simulink model "qp_torq_allocator"  (R2024b)
settings: Solver=VariableStepAuto  StartTime=0.0  StopTime=10.0  RelTol=1e-3
settings Model: Creator=lukec  LastModifiedBy=lukec

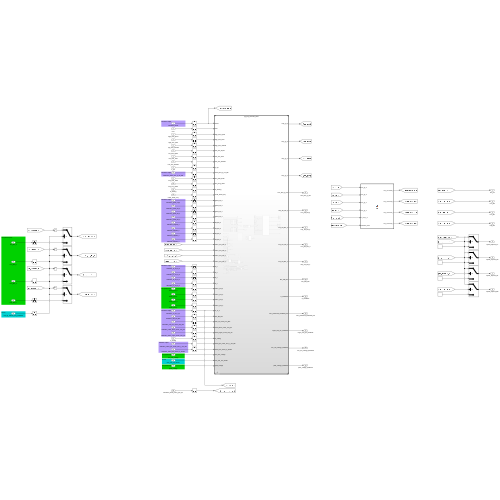
[thumbnail: Simulink's stored preview of the top-level diagram]
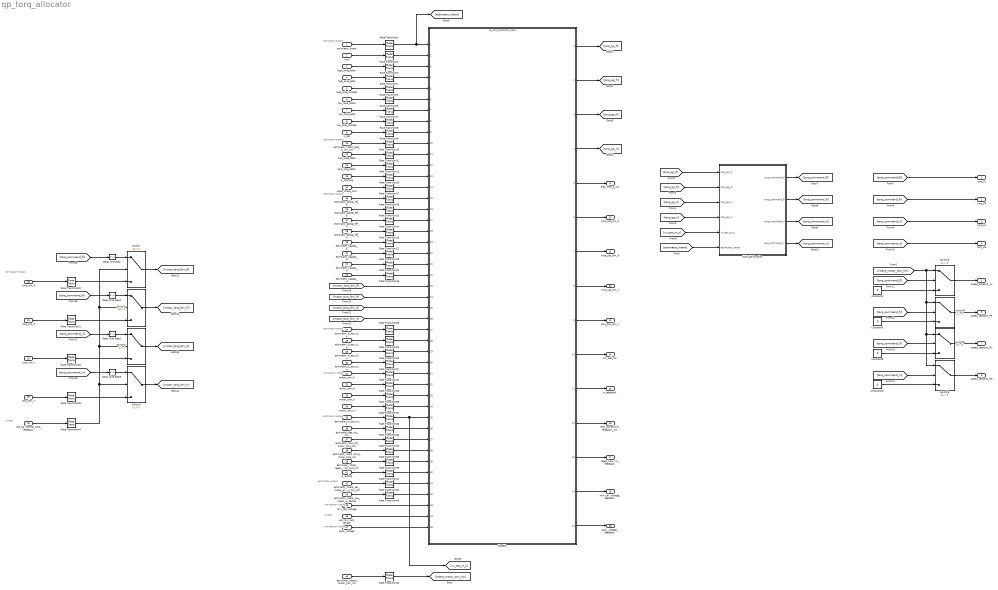
== system qp_torq_allocator ==
  note: non-param-inputs
  note: estimator-output
  note: estimator-output
  note: non-param-inputs
  note: estimator-output
  note: estimator-output
  note: estimator-output
  note: estimator-output
  note: is-bool
  note: non-param-inputs
  note: is-bool
  note: non-param-inputs
  estimator_intent : Inport
  mux : Inport  Port=2
  high_axle_alpha : Inport  Port=3
  high_axle_beta : Inport  Port=4
  high_axle_lambda : Inport  Port=5
  low_axle_alpha : Inport  Port=6
  low_axle_beta : Inport  Port=7
  low_axle_lambda : Inport  Port=8
  k_opt : Inport  Port=9
  estimator_intent_elec_p_lim_kW : Inport  Port=10
  torq_side_delta : Inport  Port=11
  torq_long_delta : Inport  Port=12
  w_starting : Inport  Port=13
  coast_brake_torq : Inport  Port=14
  estimator_global_eff_fl : Inport  Port=15
  estimator_global_eff_fr : Inport  Port=16
  estimator_global_eff_rl : Inport  Port=17
  estimator_global_eff_rr : Inport  Port=18
  estimator_kappas_fl : Inport  Port=19
  estimator_kappas_fr : Inport  Port=20
  estimator_kappas_rl : Inport  Port=21
  estimator_kappas_rr : Inport  Port=22
  torq_Nm_fl : Inport  Port=23
  torq_Nm_fr : Inport  Port=24
  torq_Nm_rl : Inport  Port=25
  torq_Nm_rr : Inport  Port=26
  estimator_fz_est_N_fl : Inport  Port=27
  estimator_fz_est_N_fr : Inport  Port=28
  estimator_fz_est_N_rl : Inport  Port=29
  estimator_fz_est_N_rr : Inport  Port=30
  motor_rpm_fl : Inport  Port=31
  motor_rpm_fr : Inport  Port=32
  motor_rpm_rl : Inport  Port=33
  motor_rpm_rr : Inport  Port=34
  estimator_vx_est_m_s : Inport  Port=35
  estimator_des_Mz_Nm : Inport  Port=36
  estimator_max_tot_motor_torq_Nm : Inport  Port=37
  estimator_intent_drive_motor_torq_lim : Inport  Port=38
  estimator_intent_regen_motor_torq_lim : Inport  Port=39
  estimator_intent_motor_rpm_lim : Inport  Port=40
  w_ending : Inport  Port=41
  estimator_intent_per_motor_elec_p_lim_kW : Inport  Port=42
  estimator_intent_use_intent_w_derate : Inport  Port=43
  use_qp_internal_torq_feedback : Inport  Port=44  OutDataTypeStr=boolean
  min_cell_voltage : Inport  Port=45
  use_min_cell_derate : Inport  Port=46  OutDataTypeStr=boolean
  pack_voltage : Inport  Port=47
  Constant{4,6,8,10} (4 alike) : Constant  Value=0
  Delay One Step{,1..3} (4 alike) : Delay  DelayLength=1  SampleTime=0.004
  MATLAB Function : MATLAB Function  TreatAsAtomicUnit=on
  Model5 : ModelReference  ModelNameDialog=qp_torq_allocator_base.slx  SimulationMode=Normal  ModelReferenceVersion=1.26
  Rate Transition{1..44} (44 alike) : RateTransition  OutPortSampleTime=0.004
  Switch{,1..7} (8 alike) : Switch  Criteria=u2 > Threshold  SaturateOnIntegerOverflow=off  InputSameDT=off
  torq_FL : Outport
  torq_FR : Outport  Port=2
  torq_RL : Outport  Port=3
  torq_RR : Outport  Port=4
  speed_setpoint_FL : Outport  Port=5
  speed_setpoint_FR : Outport  Port=6
  speed_setpoint_RL : Outport  Port=7
  speed_setpoint_RR : Outport  Port=8
  elec_theo_p_kW : Outport  Port=9
  torq_sat_Nm_fl : Outport  Port=10
  torq_sat_Nm_fr : Outport  Port=11
  torq_sat_Nm_rl : Outport  Port=12
  torq_sat_Nm_rr : Outport  Port=13
  Mz_add_Nm : Outport  Port=14
  w_feedback : Outport  Port=15
  elec_powerlimit_feedback_kW : Outport  Port=16
  regen_torq_lim_feedback : Outport  Port=17
  min_cell_voltage_feedback : Outport  Port=18
  pack_voltage_feedback : Outport  Port=19
  wires:
  estimator_intent/1 -> Rate Transition1/1
  mux/1 -> Rate Transition2/1
  high_axle_alpha/1 -> Rate Transition3/1
  high_axle_beta/1 -> Rate Transition4/1
  high_axle_lambda/1 -> Rate Transition5/1
  low_axle_alpha/1 -> Rate Transition6/1
  low_axle_beta/1 -> Rate Transition7/1
  low_axle_lambda/1 -> Rate Transition8/1
  k_opt/1 -> Rate Transition9/1
  estimator_intent_elec_p_lim_kW/1 -> Rate Transition10/1
  torq_side_delta/1 -> Rate Transition11/1
  torq_long_delta/1 -> Rate Transition12/1
  w_starting/1 -> Rate Transition16/1
  coast_brake_torq/1 -> Rate Transition17/1
  estimator_global_eff_fl/1 -> Rate Transition18/1
  estimator_global_eff_fr/1 -> Rate Transition13/1
  estimator_global_eff_rl/1 -> Rate Transition14/1
  estimator_global_eff_rr/1 -> Rate Transition15/1
  estimator_kappas_fl/1 -> Rate Transition22/1
  estimator_kappas_fr/1 -> Rate Transition23/1
  estimator_kappas_rl/1 -> Rate Transition24/1
  estimator_kappas_rr/1 -> Rate Transition19/1
  torq_Nm_fl/1 -> Rate Transition20/1
  torq_Nm_fr/1 -> Rate Transition21/1
  torq_Nm_rl/1 -> Rate Transition28/1
  torq_Nm_rr/1 -> Rate Transition29/1
  estimator_fz_est_N_fl/1 -> Rate Transition30/1
  estimator_fz_est_N_fr/1 -> Rate Transition25/1
  estimator_fz_est_N_rl/1 -> Rate Transition26/1
  estimator_fz_est_N_rr/1 -> Rate Transition27/1
  motor_rpm_fl/1 -> Rate Transition31/1
  motor_rpm_fr/1 -> Rate Transition35/1
  motor_rpm_rl/1 -> Rate Transition36/1
  motor_rpm_rr/1 -> Rate Transition37/1
  estimator_vx_est_m_s/1 -> Rate Transition32/1
  estimator_des_Mz_Nm/1 -> Rate Transition33/1
  estimator_max_tot_motor_torq_Nm/1 -> Rate Transition34/1
  estimator_intent_drive_motor_torq_lim/1 -> Rate Transition38/1
  estimator_intent_regen_motor_torq_lim/1 -> Rate Transition39/1
  Rate Transition1/1 -> [estimator_intent], Model5/1
  Rate Transition2/1 -> Model5/2
  Rate Transition3/1 -> Model5/3
  Rate Transition6/1 -> Model5/6
  Rate Transition5/1 -> Model5/5
  Rate Transition4/1 -> Model5/4
  Rate Transition8/1 -> Model5/8
  Rate Transition10/1 -> Model5/10
  Rate Transition11/1 -> Model5/11
  Rate Transition9/1 -> Model5/9
  Rate Transition12/1 -> Model5/12
  Rate Transition7/1 -> Model5/7
  Rate Transition14/1 -> Model5/17
  Rate Transition15/1 -> Model5/18
  Rate Transition16/1 -> Model5/13
  Rate Transition17/1 -> Model5/14
  Rate Transition13/1 -> Model5/16
  Rate Transition18/1 -> Model5/15
  Rate Transition19/1 -> Model5/22
  Rate Transition24/1 -> Model5/21
  Rate Transition22/1 -> Model5/19
  Rate Transition23/1 -> Model5/20
  Rate Transition26/1 -> Model5/29
  Rate Transition27/1 -> Model5/30
  Rate Transition30/1 -> Model5/27
  Rate Transition25/1 -> Model5/28
  Rate Transition31/1 -> Model5/31
  Rate Transition32/1 -> [vx_est_m_s], Model5/35
  Rate Transition33/1 -> Model5/36
  Rate Transition34/1 -> Model5/37
  Rate Transition35/1 -> Model5/32
  Rate Transition36/1 -> Model5/33
  Rate Transition37/1 -> Model5/34
  Rate Transition39/1 -> Model5/39
  Rate Transition38/1 -> Model5/38
  estimator_intent_motor_rpm_lim/1 -> Rate Transition40/1
  Rate Transition40/1 -> [intent_motor_rpm_lim]
  Model5/1 -> [torq_qp_fl]
  Model5/2 -> [torq_qp_fr]
  Model5/3 -> [torq_qp_rl]
  Model5/4 -> [torq_qp_rr]
  Constant8/1 -> Switch5/3
  Switch4/1 -> speed_setpoint_FR/1
  Switch3/1 -> speed_setpoint_FL/1
  [torq_command_fr] -> Switch4/2
  [intent_motor_rpm_lim] -> Switch6/1, Switch5/1, Switch4/1, Switch3/1
  Switch6/1 -> speed_setpoint_RR/1
  [torq_command_rr] -> Switch6/2
  Constant4/1 -> Switch3/3
  [torq_command_rl] -> Switch5/2
  Constant6/1 -> Switch4/3
  Constant10/1 -> Switch6/3
  [torq_command_fl] -> Switch3/2
  Switch5/1 -> speed_setpoint_RL/1
  Model5/5 -> elec_theo_p_kW/1
  Model5/6 -> torq_sat_Nm_fl/1
  Model5/7 -> torq_sat_Nm_fr/1
  Model5/8 -> torq_sat_Nm_rl/1
  Model5/9 -> torq_sat_Nm_rr/1
  Model5/10 -> Mz_add_Nm/1
  [torq_qp_fl] -> MATLAB Function/1(torq_qp_fl)
  [torq_qp_fr] -> MATLAB Function/2(torq_qp_fr)
  [torq_qp_rl] -> MATLAB Function/3(torq_qp_rl)
  [torq_qp_rr] -> MATLAB Function/4(torq_qp_rr)
  [vx_est_m_s] -> MATLAB Function/5(vx_est_m_s)
  [estimator_intent] -> MATLAB Function/6(estimator_intent)
  MATLAB Function/1(torq_command_fl) -> [torq_command_fl]
  MATLAB Function/2(torq_command_fr) -> [torq_command_fr]
  MATLAB Function/3(torq_command_rl) -> [torq_command_rl]
  MATLAB Function/4(torq_command_rr) -> [torq_command_rr]
  [torq_command_fl] -> torq_FL/1
  [torq_command_fr] -> torq_FR/1
  [torq_command_rl] -> torq_RL/1
  [torq_command_rr] -> torq_RR/1
  Model5/11 -> w_feedback/1
  w_ending/1 -> Rate Transition41/1
  Rate Transition42/1 -> Model5/41
  Rate Transition41/1 -> Model5/40
  estimator_intent_per_motor_elec_p_lim_kW/1 -> Rate Transition42/1
  estimator_intent_use_intent_w_derate/1 -> Rate Transition43/1
  Rate Transition43/1 -> Model5/42
  use_qp_internal_torq_feedback/1 -> Rate Transition44/1
  Rate Transition44/1 -> Switch2/2, Switch/2, Switch1/2, Switch7/2
  Rate Transition20/1 -> Switch/3
  [torq_command_fl] -> Delay One Step/1
  Delay One Step/1 -> Switch/1
  Delay One Step1/1 -> Switch1/1
  Delay One Step2/1 -> Switch2/1
  Delay One Step3/1 -> Switch7/1
  [torq_command_fr] -> Delay One Step1/1
  [torq_command_rl] -> Delay One Step2/1
  [torq_command_rr] -> Delay One Step3/1
  Rate Transition21/1 -> Switch1/3
  Rate Transition28/1 -> Switch2/3
  Rate Transition29/1 -> Switch7/3
  Model5/12 -> elec_powerlimit_feedback_kW/1
  min_cell_voltage/1 -> Model5/43
  use_min_cell_derate/1 -> Model5/44
  Model5/13 -> regen_torq_lim_feedback/1
  Switch/1 -> [motor_torq_Nm_fl]
  Switch1/1 -> [motor_torq_Nm_fr]
  Switch2/1 -> [motor_torq_Nm_rl]
  Switch7/1 -> [motor_torq_Nm_rr]
  [motor_torq_Nm_fl] -> Model5/23
  [motor_torq_Nm_fr] -> Model5/24
  [motor_torq_Nm_rr] -> Model5/26
  [motor_torq_Nm_rl] -> Model5/25
  pack_voltage/1 -> Model5/45
  Model5/14 -> min_cell_voltage_feedback/1
  Model5/15 -> pack_voltage_feedback/1

== matlab function qp_torq_allocator/MATLAB Function ==
  data: torq_qp_fl input; torq_command_fl output; torq_qp_fr input; torq_qp_rl input; torq_qp_rr input; vx_est_m_s input; torq_command_fr output; torq_command_rl output; torq_command_rr output; estimator_intent input
function [torq_command_fl, torq_command_fr, torq_command_rl, torq_command_rr] = fcn(torq_qp_fl, torq_qp_fr, torq_qp_rl, torq_qp_rr, vx_est_m_s, estimator_intent)

    regen_derate_speed = 10/3.6;
    no_regen_speed = 5/3.6;

    if vx_est_m_s < no_regen_speed
        
        % speed under 5 KPH

        if estimator_intent < 0

            % Attempting to brake, cut regen
            torq_command_fl = 0;
            torq_command_fr = 0;
            torq_command_rl = 0;
            torq_command_rr = 0;

        else

            % passthrough
            torq_command_fl = torq_qp_fl;
            torq_command_fr = torq_qp_fr;
            torq_command_rl = torq_qp_rl;
            torq_command_rr = torq_qp_rr;

        end

    elseif vx_est_m_s < regen_derate_speed && vx_est_m_s > no_regen_speed

        % speed greater than 5 KPH and less than 10 KPH

        if estimator_intent < 0

            % Attempting to brake
            gain = interp1([no_regen_speed, regen_derate_speed], [0, 1], vx_est_m_s);

            torq_command_fl = torq_qp_fl * gain;
            torq_command_fr = torq_qp_fr * gain;
            torq_command_rl = torq_qp_rl * gain;
            torq_command_rr = torq_qp_rr * gain;

        else

            % passthrough
            torq_command_fl = torq_qp_fl;
            torq_command_fr = torq_qp_fr;
            torq_command_rl = torq_qp_rl;
            torq_command_rr = torq_qp_rr;

        end

    else
        
        % speed above 10 KPH
        torq_command_fl = torq_qp_fl;
        torq_command_fr = torq_qp_fr;
        torq_command_rl = torq_qp_rl;
        torq_command_rr = torq_qp_rr;

    end
